simulink subsystem "PowerSplitHEV_DirectInput_DrvEnv_refsub"  (R2021a)
settings: Solver=VariableStepAuto  StartTime=0.0  StopTime=10.0  RelTol=1e-3
settings Model: Creator=isaacito  LastModifiedBy=isaacito
settings SolverCC: AlgebraicLoopSolver=TrustRegion
settings DebuggingCC: SFMachineParentedDataDiag=warning

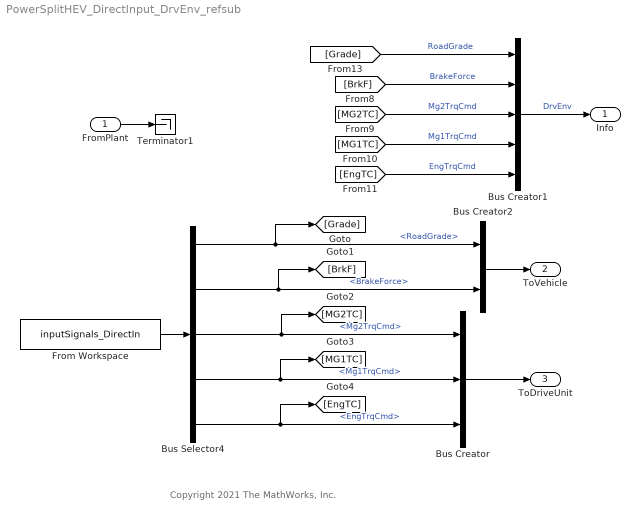
== system PowerSplitHEV_DirectInput_DrvEnv_refsub ==
  note: Copyright 2021 The MathWorks, Inc.
  FromPlant : Inport
  Bus Creator : BusCreator  Inputs=3
  Bus Creator1 : BusCreator  Inputs=5
  Bus Creator2 : BusCreator  Inputs=2
  Bus Selector4 : BusSelector  OutputSignals=RoadGrade,BrakeForce,Mg2TrqCmd,Mg1TrqCmd,EngTrqCmd
  From Workspace : FromWorkspace  VariableName=inputSignals_DirectIn  OutDataTypeStr=Bus: inputBus_DirectIn  Interpolate=off  OutputAfterFinalValue=Holding final value
      settings: AttributesFormatString=|
      | %<OutDataTypeStr>
      | Interpolate: %<Interpolate>
  Terminator1 : Terminator
  Info : Outport
  ToVehicle : Outport  Port=2
  ToDriveUnit : Outport  Port=3
  wires:
  Bus Selector4/1 -> Bus Creator2/1, [Grade]  "<RoadGrade>"
  Bus Selector4/2 -> Bus Creator2/2, [BrkF]  "<BrakeForce>"
  Bus Creator/1 -> ToDriveUnit/1
  Bus Selector4/3 -> [MG2TC], Bus Creator/1  "<Mg2TrqCmd>"
  Bus Selector4/4 -> [MG1TC], Bus Creator/2  "<Mg1TrqCmd>"
  Bus Selector4/5 -> Bus Creator/3, [EngTC]  "<EngTrqCmd>"
  From Workspace/1 -> Bus Selector4/1
  Bus Creator1/1 -> Info/1  "DrvEnv"
  [Grade] -> Bus Creator1/1  "RoadGrade"
  [BrkF] -> Bus Creator1/2  "BrakeForce"
  [MG2TC] -> Bus Creator1/3  "Mg2TrqCmd"
  [MG1TC] -> Bus Creator1/4  "Mg1TrqCmd"
  [EngTC] -> Bus Creator1/5  "EngTrqCmd"
  FromPlant/1 -> Terminator1/1
  Bus Creator2/1 -> ToVehicle/1
